simulink model "Three_Phase_SPWM_BucK_rectifier2015b"  (Simulink 8.6)
settings: Solver=ode45  StartTime=0.0  StopTime=3  RelTol=1e-3
libraries: powerlib x31, simulink x2
settings Model: Creator=sample  LastModifiedBy=A0109971
settings DebuggingCC: FcnCallInpInsideContextMsg=EnableAllAsWarning  AllowSymbolicDim=on

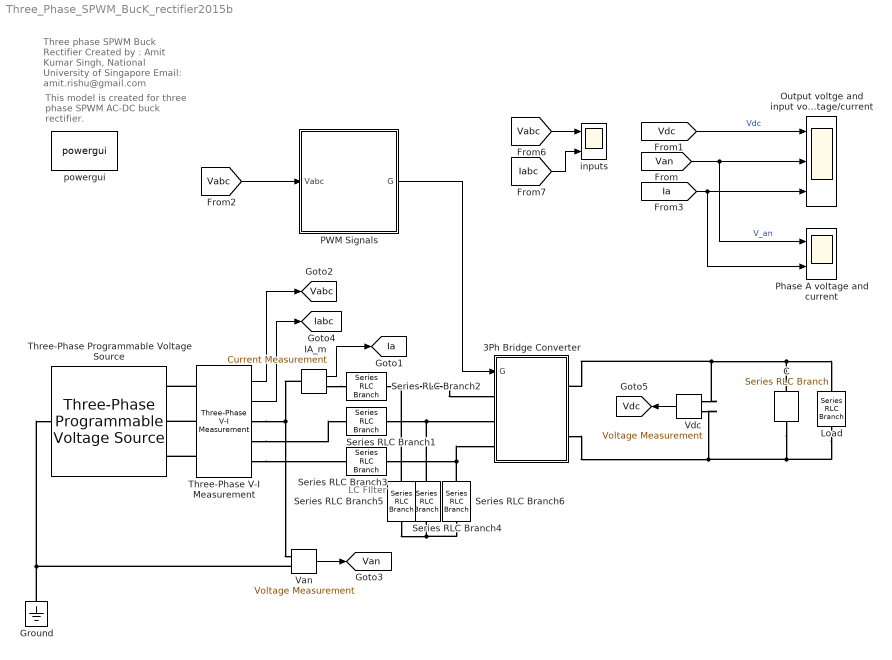
== system Three_Phase_SPWM_BucK_rectifier2015b ==
  note: This model is created for three phase SPWM AC-DC buck rectifier.
  note: Three phase SPWM Buck Rectifier
      |
      | Created by : Amit Kumar Singh, National University of Singapore
      | Email: amit.rishu@gmail.com
  note: LC FIlter
  3Ph Bridge Converter : Subsystem
  C : powerlib/Elements/Series RLC Branch  LConnTagsString=__new0  RConnTagsString=__new0  BranchType=C  Resistance=1  Inductance=1e-3  SetiL0=off  InitialCurrent=0  Capacitance=1000e-6  Setx0=off  InitialVoltage=0  Measurements=None
  Ground : powerlib/Elements/Ground  LConnTagsString=a
  IA_m : powerlib/Measurements/Current Measurement  PhasorSimulation=off  OutputType=Complex  PSBequivalent=0
  Load : powerlib/Elements/Series RLC Branch  LConnTagsString=__new0  RConnTagsString=__new0  BranchType=R  Resistance=10  Inductance=1e-3  SetiL0=off  InitialCurrent=0  Capacitance=0  Setx0=off  InitialVoltage=0  Measurements=None
  Output voltge and input voltage/current : Scope  NumInputPorts=3
  PWM Signals : Subsystem
  Phase A voltage and current : Scope  NumInputPorts=2
  Series RLC Branch1 : powerlib/Elements/Series RLC Branch  LConnTagsString=__new0  RConnTagsString=__new0  BranchType=L  Resistance=.1  Inductance=1e-3  SetiL0=off  InitialCurrent=0  Capacitance=200e-6  Setx0=off  InitialVoltage=0  Measurements=None
  Series RLC Branch2 : powerlib/Elements/Series RLC Branch  LConnTagsString=__new0  RConnTagsString=__new0  BranchType=L  Resistance=0.1  Inductance=1e-3  SetiL0=off  InitialCurrent=0  Capacitance=200e-6  Setx0=off  InitialVoltage=0  Measurements=None
  Series RLC Branch3 : powerlib/Elements/Series RLC Branch  LConnTagsString=__new0  RConnTagsString=__new0  BranchType=L  Resistance=0.1  Inductance=1e-3  SetiL0=off  InitialCurrent=0  Capacitance=200e-6  Setx0=off  InitialVoltage=0  Measurements=None
  Series RLC Branch4 : powerlib/Elements/Series RLC Branch  LConnTagsString=__new0  RConnTagsString=__new0  BranchType=C  Resistance=0.1  Inductance=1e-3  SetiL0=off  InitialCurrent=0  Capacitance=20e-6  Setx0=off  InitialVoltage=0  Measurements=None
  Series RLC Branch5 : powerlib/Elements/Series RLC Branch  LConnTagsString=__new0  RConnTagsString=__new0  BranchType=C  Resistance=0.1  Inductance=1e-3  SetiL0=off  InitialCurrent=0  Capacitance=20e-6  Setx0=off  InitialVoltage=0  Measurements=None
  Series RLC Branch6 : powerlib/Elements/Series RLC Branch  LConnTagsString=__new0  RConnTagsString=__new0  BranchType=C  Resistance=0.1  Inductance=1e-3  SetiL0=off  InitialCurrent=0  Capacitance=20e-6  Setx0=off  InitialVoltage=0  Measurements=None
  Three-Phase Programmable Voltage Source : powerlib/Electrical Sources/Three-Phase Programmable Voltage Source  PositiveSequence="[230*1.732  0 50]"  VariationEntity=None  VariationType=Table of time-amplitude pairs  VariationTypeAlt=Step  VariationStep=0.5  VariationRate=10  VariationMagnitude=0.3  VariationFrequency=2  VariationTiming=[1 2]  VariationPhaseA=off  Amplitudes=[1 0.8 1.2 1.0]  TimeValues=[0 0.1 0.15 0.2]  HarmonicGeneration=off  HarmonicA=[3 0.2 -25 0]  HarmonicB=[2 0.15 35 2]  Timing="[0.05  3]"  BusType=swing  Pref=0  Qref=0  Qmin=-inf  Qmax=inf
  Three-Phase V-I Measurement : powerlib/Measurements/Three-Phase V-I Measurement  VoltageMeasurement=phase-to-ground  SetLabelV=off  LabelV=Vabc  Vpu=off  VpuLL=off  CurrentMeasurement=yes  SetLabelI=off  LabelI=Iabc  Ipu=off  Pbase=100e6  Vbase=500e3  OutputType=Complex  PhasorSimulation=off  PSBequivalent=0
  Van : powerlib/Measurements/Voltage Measurement  Tag=PoWeRsYsTeMmEaSuReMeNt  PhasorSimulation=off  OutputType=Magnitude  PSBequivalent=0
  "Vdc " : powerlib/Measurements/Voltage Measurement  Tag=PoWeRsYsTeMmEaSuReMeNt  PhasorSimulation=off  OutputType=Magnitude  PSBequivalent=0
  inputs : Scope  NumInputPorts=2
  powergui : powerlib/powergui  Priority=1  SimulationMode=Discrete  SampleTime=2e-6  frequency=60  Iterations=50  frequencyindice=0  Pbase=100e6  ErrMax=1e-4  UnitsV=kV  UnitsW=MW  buscounter=0  FunctionMessages=off  echomessages=off  EnableUseOfTLC=off  CurrentSourceSwitches=off  DisableSnubberDevices=off  DisableRonSwitches=off  DisableVfSwitches=off  DisplayEquations=off  SolverType=Tustin  Interpol=off  ExternalGateDelay=off  methode=off  Ts=100  x0status=blocks  SPID=off  SwTol=0  HookPort=off  RestoreLinks=warning  ResistiveCurrentMeasurement=off  Frange=[0:2:500]  Ylog=off  Xlog=on  ShowGrid=off  save=off  variable=ZData  structure=ScopeData  ZoomFFT=off  StartTime=0.6  cycles=4  DisplayStyle=4  fundamental=50  FreqAxis=on  MaxFrequency=650  frequencyindicesteady=1  RmsSteady=1  display=off
  tag scope: Ia=global, Iabc=global, Vabc=global, Van=global, Vdc=global
  wires:
  [Van] -> Phase A voltage and current/1, Output voltge and input voltage/current/2  "V_an"
  "Vdc "/1 -> [Vdc]
  [Vdc] -> Output voltge and input voltage/current/1  "Vdc"
  Van/1 -> [Van]
  IA_m/1 -> [Ia]
  Three-Phase V-I Measurement/1 -> [Vabc]
  Three-Phase V-I Measurement/2 -> [Iabc]
  PWM Signals/1(G) -> 3Ph Bridge Converter/1(G)
  [Ia] -> Phase A voltage and current/2, Output voltge and input voltage/current/3
  [Vabc] -> inputs/1
  [Iabc] -> inputs/2
  [Vabc] -> PWM Signals/1(Vabc)
  connections:
  Load/RConn1 -- C/RConn1 -- "Vdc "/LConn2 -- 3Ph Bridge Converter/RConn2
  IA_m/LConn1 -- Three-Phase V-I Measurement/RConn1 -- Van/LConn1
  "Vdc "/LConn1 -- C/LConn1 -- Load/LConn1 -- 3Ph Bridge Converter/RConn1
  Series RLC Branch2/LConn1 -- Series RLC Branch5/LConn1 -- 3Ph Bridge Converter/LConn1
  Series RLC Branch1/LConn1 -- Series RLC Branch4/LConn1 -- 3Ph Bridge Converter/LConn2
  Series RLC Branch3/LConn1 -- Series RLC Branch6/LConn1 -- 3Ph Bridge Converter/LConn3
  Van/LConn2 -- Three-Phase Programmable Voltage Source/LConn1 -- Ground/LConn1
  IA_m/RConn1 -- Series RLC Branch2/RConn1
  Three-Phase V-I Measurement/LConn1 -- Three-Phase Programmable Voltage Source/RConn1
  Three-Phase V-I Measurement/LConn2 -- Three-Phase Programmable Voltage Source/RConn2
  Three-Phase V-I Measurement/LConn3 -- Three-Phase Programmable Voltage Source/RConn3
  Three-Phase V-I Measurement/RConn2 -- Series RLC Branch1/RConn1
  Three-Phase V-I Measurement/RConn3 -- Series RLC Branch3/RConn1
  Series RLC Branch5/RConn1 -- Series RLC Branch6/RConn1 -- Series RLC Branch4/RConn1

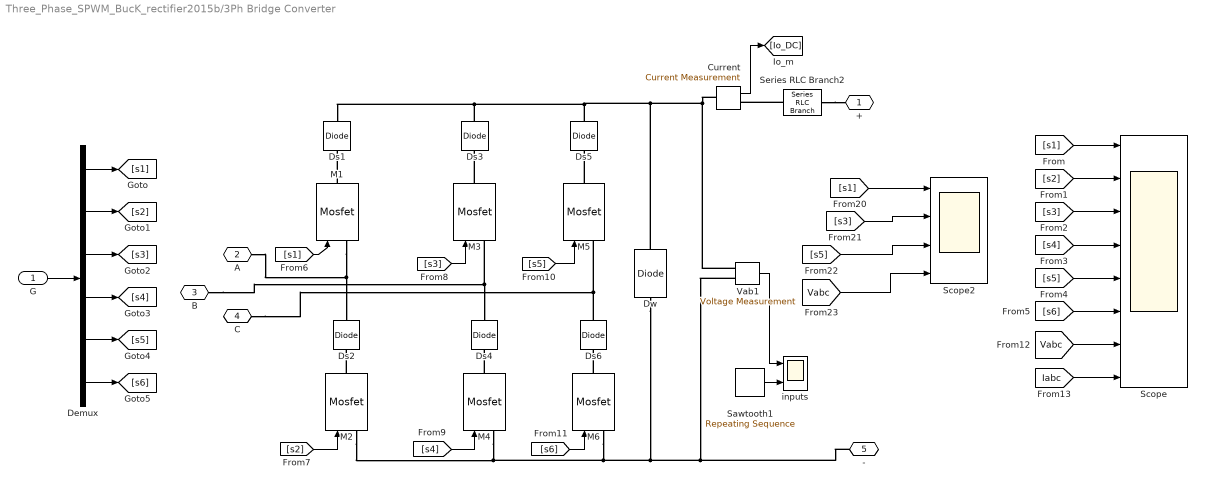
== system Three_Phase_SPWM_BucK_rectifier2015b/3Ph Bridge Converter ==
  G : Inport
  Current : powerlib/Measurements/Current Measurement  PhasorSimulation=off  OutputType=Complex  PSBequivalent=0
  Demux : Demux  Outputs=6
  Ds{1..6} (6 alike) : powerlib/Power Electronics/Diode  Ron=0.0001  Lon=0  Vf=0  IC=0  UseSnubber=off  Rs=5000  Cs=250e-9  Measurements=off
  Dw : powerlib/Power Electronics/Diode  Ron=0.0001  Lon=0  Vf=0  IC=0  UseSnubber=off  Rs=5000  Cs=250e-9  Measurements=off
  M{1..6} (6 alike) : powerlib/Power Electronics/Mosfet  Ron=0.1  Lon=0  Rd=0.01  Vfd=0  IC=0  Rs=1e5  Cs=inf  Measurements=off
  Sawtooth1 : simulink/Sources/Repeating Sequence  rep_seq_t=[0 1/10e3]  rep_seq_y=[0 1]
  Scope : Scope  NumInputPorts=8
  Scope2 : Scope  NumInputPorts=4
  Series RLC Branch2 : powerlib/Elements/Series RLC Branch  LConnTagsString=__new0  RConnTagsString=__new0  BranchType=L  Resistance=0.1  Inductance=2.5e-3  SetiL0=off  InitialCurrent=0  Capacitance=200e-6  Setx0=off  InitialVoltage=0  Measurements=None
  Vab1 : powerlib/Measurements/Voltage Measurement  Tag=PoWeRsYsTeMmEaSuReMeNt  PhasorSimulation=off  OutputType=Magnitude  PSBequivalent=0
  inputs : Scope  NumInputPorts=2
  + : PMIOPort  Port=1  Side=Right
  A : PMIOPort  Port=2  Side=Left
  B : PMIOPort  Port=3  Side=Left
  C : PMIOPort  Port=4  Side=Left
  - : PMIOPort  Port=5  Side=Right
  wires:
  [s2] -> M2/1
  [s3] -> M3/1
  [s4] -> M4/1
  Demux/1 -> [s1]
  Demux/2 -> [s2]
  Demux/3 -> [s3]
  Demux/4 -> [s4]
  Demux/5 -> [s5]
  Demux/6 -> [s6]
  G/1 -> Demux/1
  Current/1 -> [Io_DC]
  [s1] -> Scope/1
  [s2] -> Scope/2
  [s3] -> Scope/3
  [s4] -> Scope/4
  [s5] -> Scope/5
  [s6] -> Scope/6
  [Vabc] -> Scope/7
  [Iabc] -> Scope/8
  [s1] -> Scope2/1
  [s3] -> Scope2/2
  [s5] -> Scope2/3
  [Vabc] -> Scope2/4
  [s1] -> M1/1
  [s5] -> M5/1
  [s6] -> M6/1
  Vab1/1 -> inputs/1
  Sawtooth1/1 -> inputs/2
  connections:
  Ds3/RConn1 -- Vab1/LConn1 -- Current/LConn1 -- Dw/RConn1 -- Ds5/RConn1 -- Ds1/RConn1
  -/RConn1 -- Vab1/LConn2 -- Dw/LConn1 -- M6/LConn1 -- M2/LConn1 -- M4/LConn1
  M2/RConn1 -- Ds2/LConn1
  C/RConn1 -- M5/LConn1 -- Ds6/RConn1
  A/RConn1 -- M1/LConn1 -- Ds2/RConn1
  M3/RConn1 -- Ds3/LConn1
  B/RConn1 -- Ds4/RConn1 -- M3/LConn1
  M5/RConn1 -- Ds5/LConn1
  Series RLC Branch2/RConn1 -- Current/RConn1
  Series RLC Branch2/LConn1 -- +/RConn1
  M1/RConn1 -- Ds1/LConn1
  M4/RConn1 -- Ds4/LConn1
  M6/RConn1 -- Ds6/LConn1

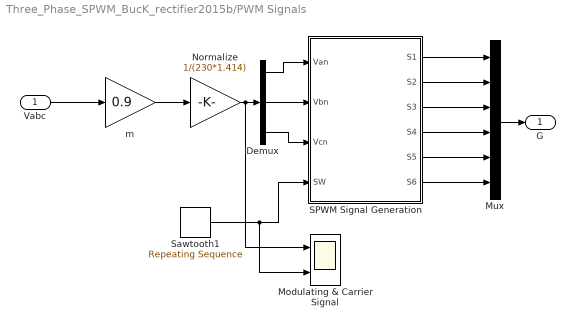
== system Three_Phase_SPWM_BucK_rectifier2015b/PWM Signals ==
  Vabc : Inport
  Demux : Demux  Outputs=3
  "Modulating & Carrier Signal " : Scope  NumInputPorts=2
  Mux : Mux  Inputs=6
  Normalize : Gain  Gain=1/(230*1.414)
  SPWM Signal Generation : MATLAB Function  TreatAsAtomicUnit=on
  Sawtooth1 : simulink/Sources/Repeating Sequence  rep_seq_t=[0 1/10e3]  rep_seq_y=[0 1]
  m : Gain  Gain=0.9
  G : Outport
  wires:
  Demux/1 -> SPWM Signal Generation/1(Van)
  Demux/3 -> SPWM Signal Generation/3(Vcn)
  Sawtooth1/1 -> "Modulating & Carrier Signal "/2, SPWM Signal Generation/4(SW)
  Demux/2 -> SPWM Signal Generation/2(Vbn)
  SPWM Signal Generation/1(S1) -> Mux/1
  SPWM Signal Generation/2(S2) -> Mux/2
  SPWM Signal Generation/3(S3) -> Mux/3
  SPWM Signal Generation/4(S4) -> Mux/4
  SPWM Signal Generation/5(S5) -> Mux/5
  SPWM Signal Generation/6(S6) -> Mux/6
  Vabc/1 -> m/1
  Mux/1 -> G/1
  Normalize/1 -> "Modulating & Carrier Signal "/1, Demux/1
  m/1 -> Normalize/1

== matlab function PWM Signals/SPWM Signal Generation ==
  data: Van input double; S1 output double; Vbn input double; Vcn input double; SW input double; S2 output double; S3 output double; S4 output double; S5 output double; S6 output double
%% Switching Signal Generation for Buck Rectifier
%The three phase input voltages are sensed and given to controller.
% With Saw-tooth singal of required switching frequency, the SPWM 
%switching signal S1-S6 are generated.
function [S1,S2,S3,S4,S5,S6] = fcn(Van,Vbn,Vcn, SW)
%Default Switch State
S1 = false;
S2 = false;
S3 = false;
S4 = false;
S5 = false;
S6 = false;
%% Here, input voltage are divided into six sectors
% sector- 1
if (Van > 0 && Vbn <0 && Vcn < 0)
    S1 = true;
    S4 = abs(Vbn) > SW;
    S6 = and (abs(Vcn+Vbn) > SW, not(S4));
end
% sector- 2
if (Vcn < 0 && Vbn > 0 && Van > 0)
    S6 = true;
    S1 = abs(Van) >SW;
    S3 = and (abs(Van+Vbn) > SW, not(S1));
end
% sector- 3
if (Vbn > 0 && Van <0 && Vcn < 0)
    S3 = true;
    S2 = abs(Van) > SW;
    S6 = and (abs(Vcn+Van) > SW, not(S2));
end
% sector-4
if (Van < 0 && Vbn > 0 && Vcn > 0)
    S2 = true;
    S3 = abs(Vbn) > SW;
    S5 = and (abs(Vbn+Vcn) > SW, not(S3)); 
end
% sector- 5
if (Vcn > 0 && Van <0 && Vbn < 0)
    S5 = true;
    S2 = abs(Van) > SW;
    S4 = and (abs(Vbn+Van) > SW, not(S2));
end
% sector- 6
if (Vbn< 0 && Van > 0 && Vcn > 0)
    S4 = true;
    S1 = abs(Van) > SW;
    S5 = and (abs(Vcn+Van) > SW, not(S1));
end
